simulink model "RBNN_NNT_timing_of_learning_1layerRBNN_openloop"  (R2019a)
settings: Solver=FixedStepAuto  StartTime=0.0  StopTime=inf  FixedStep=0.000001  RelTol=1e-3
libraries: dspstat3 x6, dspxfrm3 x1
(part 3 of 3)

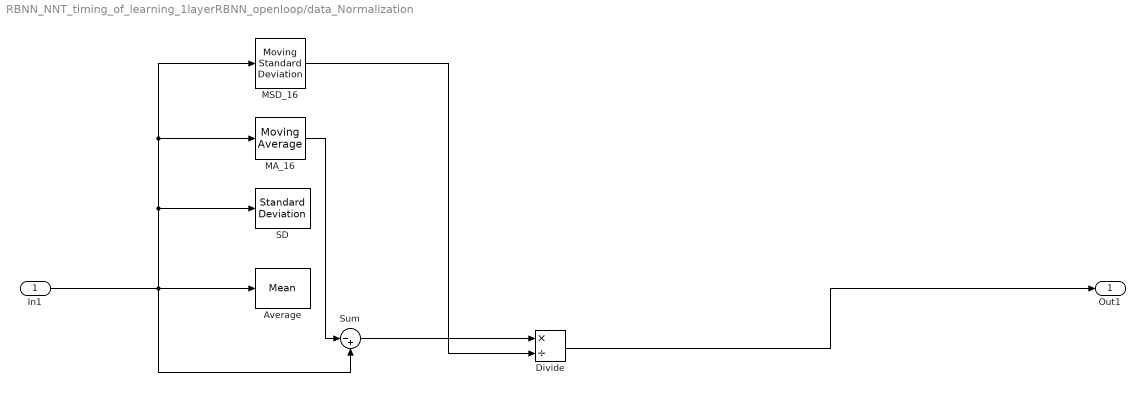
== system RBNN_NNT_timing_of_learning_1layerRBNN_openloop/data_Normalization ==
  In1 : Inport
  Average : dspstat3/Mean  run=on  reset_popup=None  directionMode=Each column  dimension=1  roiEnable=off  roiType=Rectangles  roiPortion=Entire ROI  roiOutput=Individual statistics for each ROI  roiFlag=off  roundingMode=Floor  overflowMode=off  outputDataTypeStr=Inherit: Same as accumulator  outputMin=[]  outputMax=[]  outputLastDataTypeStr=Inherit: Same as accumulator
  Divide : Product  Inputs=*/
  MA_16 : dspstat3/Moving Average  Method=Sliding window  ForgettingFactorPort=off  SpecifyWindowLength=on  WindowLength=4  ForgettingFactor=0.9  SimulateUsing=Code generation
  MSD_16 : dspstat3/Moving Standard Deviation  Method=Sliding window  ForgettingFactorPort=off  SpecifyWindowLength=on  WindowLength=4  ForgettingFactor=0.9  SimulateUsing=Code generation
      settings: SourceProductName=DSP System Toolbox  SourceProductBaseCode=DS
  SD : dspstat3/Standard Deviation  run=on  directionMode=Each column  dimension=1  reset_popup=None  roiEnable=off  roiType=Rectangles  roiPortion=Entire ROI  roiOutput=Individual statistics for each ROI  roiFlag=off
      settings: SourceProductName=DSP System Toolbox  SourceProductBaseCode=DS
  Sum : Sum  Inputs=|-+
  Out1 : Outport
  wires:
  In1/1 -> Sum/2, SD/1, MA_16/1, MSD_16/1, Average/1
  Sum/1 -> Divide/1
  Divide/1 -> Out1/1
  MSD_16/1 -> Divide/2
  MA_16/1 -> Sum/1

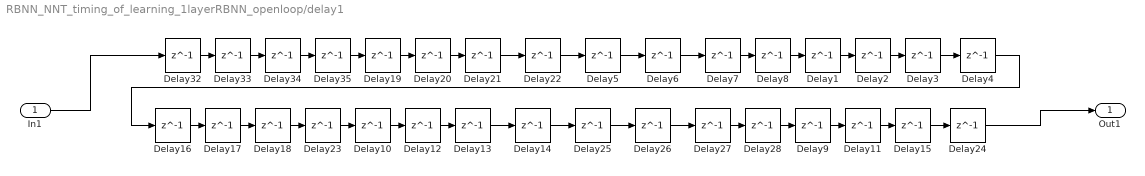
== system RBNN_NNT_timing_of_learning_1layerRBNN_openloop/delay1 ==
  In1 : Inport
  Delay{1..28,32..35} (32 alike) : Delay  DelayLength=1  InitialCondition=0
  Out1 : Outport
  wires:
  Delay34/1 -> Delay35/1
  Delay35/1 -> Delay19/1
  Delay33/1 -> Delay34/1
  Delay20/1 -> Delay21/1
  Delay21/1 -> Delay22/1
  Delay19/1 -> Delay20/1
  Delay32/1 -> Delay33/1
  Delay7/1 -> Delay8/1
  Delay8/1 -> Delay1/1
  Delay6/1 -> Delay7/1
  Delay2/1 -> Delay3/1
  Delay3/1 -> Delay4/1
  Delay1/1 -> Delay2/1
  Delay5/1 -> Delay6/1
  Delay22/1 -> Delay5/1
  Delay18/1 -> Delay23/1
  Delay15/1 -> Delay24/1
  Delay10/1 -> Delay12/1
  Delay17/1 -> Delay18/1
  Delay16/1 -> Delay17/1
  Delay13/1 -> Delay14/1
  Delay25/1 -> Delay26/1
  Delay27/1 -> Delay28/1
  Delay28/1 -> Delay9/1
  Delay14/1 -> Delay25/1
  Delay11/1 -> Delay15/1
  Delay26/1 -> Delay27/1
  Delay9/1 -> Delay11/1
  Delay23/1 -> Delay10/1
  Delay12/1 -> Delay13/1
  Delay4/1 -> Delay16/1
  Delay24/1 -> Out1/1
  In1/1 -> Delay32/1

== matlab function RBNN_NNT_timing_of_learning_1layerRBNN_openloop/NNT_O32 ==
  settings: sampleTime=0.125
  data: X0 input; X1 input; X2 input; X3 input; X4 input; X5 input; X6 input; X7 input; X8 input; X9 input; X10 input; X11 input; X12 input; X13 input; X14 input; X15 input; df input; y output; cost output; stop input; alpha_l input; a input
function [y,cost] = NN(X0,X1,X2,X3,X4,X5,X6,X7,X8,X9,X10,X11,X12,X13,X14,X15,df,stop,alpha_l,a)

%This is a generalised code for 2 layer - multiple input-single output network.
% to alter the network (1) "change layer's size" in layer declaration below (2) the function
%input and output above and (3) Input matrix creation. (4) change inputs in
%simulink design

alpha = alpha_l;

%(1)layer decalration

layer_0= 17;  % make it "16 + external_input's size"
layer_1=32;
layer_2 =1;


%(2) is above in function block

%(3)parameter intialisation
v=[X0 X1 X2 X3 X4 X5 X6 X7 X8 X9 X10 X11 X12 X13 X14 X15 transpose(a)];

%Do not alter the code below. The below implementaion is generalised for
%multiple input and single output, 2 layer neural network. 


persistent w1 w2;
persistent a1 a2;
persistent J; 
persistent v_old; 

if isempty(a1)
    a1= zeros(layer_1,1);
end

if isempty(a2)
    a2= zeros(layer_2,1);
end


if isempty(J)
    J= 0;
end
if isempty(v_old)
    v_old= zeros(1,layer_0);
end



if isempty(w1)
       w1=randn(layer_1,layer_0);
end
if isempty(w2)
       w2=randn(layer_2,layer_1);
end

%BackProp:
if stop==0
dz2=a2.*(1-a2)*df*-1;
dw2=dz2*transpose(a1);
dz1=(a1.*(1-a1)).*(w2'*dz2);
%dz1=a1.*(1-a1)*dz2;
dw1=dz1*v;
w2=w2 + alpha*dw2;
w1=w1 + alpha*dw1;
v_old=v;
end 

%forward propogation
z1=w1*v';
a1= (1./(1+exp(-z1)));
an1=a1-0.5;
z2=w2*an1;
a2= (1./(1+exp(-z2)));
an2=a2-0.5;
cost=1/2*df^2;

%output assignment
y=an2;


end

== matlab function RBNN_NNT_timing_of_learning_1layerRBNN_openloop/NN_RBNN_NN ==
  settings: sampleTime=0.01
  data: u1 input; df input; F input; u2 input; nn_op output; weights output; cost output; z1_out output; stop input; alp input; grad output; df_out output; del_weights output
function [nn_op,weights,cost,z1_out,grad,df_out,del_weights]   = NN(u1,df,F,u2,stop,alp)

persistent w1 ;
persistent vy;
persistent g1 ;
persistent itr;
persistent J;
persistent del_w1 ;
persistent mult1 ;
persistent memory_alloc_flag;
persistent n;

%%
%%%%%%----------------------------------------------------------------------------%%%%%
%Hyper-parameter & other tunable part of code

M=16;   %declare batch size of training (It will also be equal to number of input in our case as we are using DFT)
E=1;    % size of external associative input

%layer declaration
layer_1=16;
      % Output layer must match with number of rezonators declared in rezonator function

%learning rate. Currently reading from input pin 
alpha = alp;

%others
input_layer =M+E;       %layer_0
output_layer=layer_1;

% weight Intialisation 
if isempty(w1)
       w1=randn(input_layer,layer_1)*0.1;
end


%%%%%---------------------------------------------------------------------------------%%%%%

%%

%synchronising clock
if isempty(n)
        n = 0; end
n=n+1;

%%
%Allocation of variables that will be used during runtime( one time execution code) 
if isempty(memory_alloc_flag)
        memory_alloc_flag = 0; 
end
if isempty(mult1)
       mult1=zeros(layer_1,layer_1*input_layer); 
end
if isempty(vy)
       vy=zeros(input_layer,M); 
end

if memory_alloc_flag==0
 %write memory allocation for looped code here.It runs once and store it in memory.  
 mult1=[];
  for iteration =1:layer_1
   mult1=[mult1;[zeros(1,(iteration-1)*input_layer) ones(1,input_layer) zeros(1,(layer_1-iteration)*input_layer)]];
  end
  
 %{
 for k= 1:input_layer
    for j = 1:M 
        if k<=(M/2)+1 && k>=1
            vy(k,j)=0;
        elseif k<=M && k>=(M/2)+1
            vy(k,j)=0;
        elseif k>M
            vy(k,j)=0;     
        end
    end
 end
  %}
 memory_alloc_flag=1; 
end

%%
%============All other Initiaisation =========================>

%Initialisation of delta of weight storage
if isempty(del_w1)
    del_w1=zeros(1,input_layer*layer_1);
end


%Intialising iteration number & cost value. 
if isempty(itr)
    itr=0;
end
if isempty(J)
    J=0;
end


%gradient initialisation(in matrix form)
if isempty(g1)
    g1= zeros(M,input_layer*layer_1);   
end


%%
%Input vector creation code block
%x_in = [real(u1(1:(size(u1,2)/2)+1)) imag(u1(1:(size(u1,2)/2)-1))];
x_in=u1';
v=transpose([x_in transpose(u2)]);

%%
%RBNN core vectorised algorithm implementation 

%--------------->forward propogation ------------>

z1=w1'*v ;
a1=(1./(1+exp(-z1)));
an1=(a1-0.5);

%-------------> Backward Propogation -------->

%calculation of Nv:
da1_z1=a1.*(1-a1);
dn_a1=w1'.*repmat(da1_z1,1,size(v,1));
 

%calculation of aD, A & B 
aD=transpose(F)*dn_a1*vy;
A=[aD;eye(M-1) zeros(M-1,1)];
B=[transpose(F) ; zeros(M-1,size(F,1))]; 

%calculation of Nw(diff of N(v,w) wrt each weights)
dIn_1= da1_z1*transpose(v);
dn_w1=repmat(dIn_1,1,layer_1).* mult1;


%gradient updation

g1=A*g1+B*dn_w1;

%Training & updation only once in a batch(batch size=M,n=Overall counter) 
if mod(n,M)==0 && stop==0
%if stop==0
    %del_w1 =alpha*df(1)*1*g1(1,:) ;
    del_w1 =alpha*df*1*g1/M ;
    del_w_reshaped1= reshape(del_w1,[input_layer,layer_1]);
    w1=w1+ del_w_reshaped1;
    itr=itr+1;
    %J= sum(df.^2,'all')/(2*M);
end

J= 1/2*df(1).^2;
%For logging & visulisation purpose
cost=J;
weights=w1;
z1_out=z1;
grad=g1(1,:);
df_out=df(1);
del_weights=del_w1;
%NN output assignment
nn_op=an1;


end

== matlab function RBNN_NNT_timing_of_learning_1layerRBNN_openloop/buffer_of_op_fft ==
  data: output_difference_vector output size=[1,16]; output_fft output size=[1,16]; dif_ip input; rbnn_output input
function [output_difference_vector,output_fft] = difBuffer(dif_ip,rbnn_output)                      

 sz=16;                       % size of the dft 
 
 persistent a;
 persistent b;
 if isempty(b)
  b= zeros(1,sz);
 end
 if isempty(a)
  a= zeros(1,sz);
 end
 
 
  a= circshift(a,1);
  a(1)=dif_ip;
  b= circshift(b,1);
  b(1)=rbnn_output;

 output_difference_vector=a; 
 output_fft=1/sz*fft(b); 
end

== matlab function RBNN_NNT_timing_of_learning_1layerRBNN_openloop/NNT_O64 ==
  settings: sampleTime=0.125
  data: X0 input; X1 input; X2 input; X3 input; X4 input; X5 input; X6 input; X7 input; X8 input; X9 input; X10 input; X11 input; X12 input; X13 input; X14 input; X15 input; df input; y output; cost output; stop input; alpha_l input; a input
function [y,cost] = NN(X0,X1,X2,X3,X4,X5,X6,X7,X8,X9,X10,X11,X12,X13,X14,X15,df,stop,alpha_l,a)

%This is a generalised code for 2 layer - multiple input-single output network.
% to alter the network (1) "change layer's size" in layer declaration below (2) the function
%input and output above and (3) Input matrix creation. (4) change inputs in
%simulink design

alpha = alpha_l;

%(1)layer decalration

layer_0= 17;  % make it "16 + external_input's size"
layer_1=64;
layer_2 =1;


%(2) is above in function block

%(3)parameter intialisation
v=[X0 X1 X2 X3 X4 X5 X6 X7 X8 X9 X10 X11 X12 X13 X14 X15 transpose(a)];

%Do not alter the code below. The below implementaion is generalised for
%multiple input and single output, 2 layer neural network. 


persistent w1 w2;
persistent a1 a2;
persistent J; 
persistent v_old; 

if isempty(a1)
    a1= zeros(layer_1,1);
end

if isempty(a2)
    a2= zeros(layer_2,1);
end


if isempty(J)
    J= 0;
end
if isempty(v_old)
    v_old= zeros(1,layer_0);
end



if isempty(w1)
       w1=randn(layer_1,layer_0);
end
if isempty(w2)
       w2=randn(layer_2,layer_1);
end

%BackProp:
if stop==0
dz2=a2.*(1-a2)*df*-1;
dw2=dz2*transpose(a1);
dz1=(a1.*(1-a1)).*(w2'*dz2);
%dz1=a1.*(1-a1)*dz2;
dw1=dz1*v;
w2=w2 + alpha*dw2;
w1=w1 + alpha*dw1;
v_old=v;
end 

%forward propogation
z1=w1*v';
a1= (1./(1+exp(-z1)));
an1=a1-0.5;
z2=w2*an1;
a2= (1./(1+exp(-z2)));
an2=a2-0.5;
cost=1/2*df^2;

%output assignment
y=an2;


end

== matlab function RBNN_NNT_timing_of_learning_1layerRBNN_openloop/NNT_O16 ==
  settings: sampleTime=0.125
  data: X0 input; X1 input; X2 input; X3 input; X4 input; X5 input; X6 input; X7 input; X8 input; X9 input; X10 input; X11 input; X12 input; X13 input; X14 input; X15 input; df input; y output; cost output; stop input; alpha_l input; a input
function [y,cost] = NN(X0,X1,X2,X3,X4,X5,X6,X7,X8,X9,X10,X11,X12,X13,X14,X15,df,stop,alpha_l,a)

%This is a generalised code for 2 layer - multiple input-single output network.
% to alter the network (1) "change layer's size" in layer declaration below (2) the function
%input and output above and (3) Input matrix creation. (4) change inputs in
%simulink design

alpha = alpha_l;

%(1)layer decalration

layer_0= 17;  % make it "16 + external_input's size"
layer_1=16;
layer_2 =1;


%(2) is above in function block

%(3)parameter intialisation
v=[X0 X1 X2 X3 X4 X5 X6 X7 X8 X9 X10 X11 X12 X13 X14 X15 transpose(a)];

%Do not alter the code below. The below implementaion is generalised for
%multiple input and single output, 2 layer neural network. 


persistent w1 w2;
persistent a1 a2;
persistent J; 
persistent v_old; 

if isempty(a1)
    a1= zeros(layer_1,1);
end

if isempty(a2)
    a2= zeros(layer_2,1);
end


if isempty(J)
    J= 0;
end
if isempty(v_old)
    v_old= zeros(1,layer_0);
end



if isempty(w1)
       w1=randn(layer_1,layer_0);
end
if isempty(w2)
       w2=randn(layer_2,layer_1);
end

%BackProp:
if stop==0
dz2=a2.*(1-a2)*df*-1;
dw2=dz2*transpose(a1);
dz1=(a1.*(1-a1)).*(w2'*dz2);
%dz1=a1.*(1-a1)*dz2;
dw1=dz1*v;
w2=w2 + alpha*dw2;
w1=w1 + alpha*dw1;
v_old=v;
end 

%forward propogation
z1=w1*v';
a1= (1./(1+exp(-z1)));
an1=a1-0.5;
z2=w2*an1;
a2= (1./(1+exp(-z2)));
an2=a2-0.5;
cost=1/2*df^2;

%output assignment
y=an2;


end

== matlab function RBNN_NNT_timing_of_learning_1layerRBNN_openloop/software_rezonator ==
  data: signalz input; reconstructed_signal output; Fn output size=16
function [reconstructed_signal,Fn]   = rezonator(signalz)

persistent numberofrezonator;
persistent g c bfr_rezo_sm aft_delay dft_out;
persistent out signal_dif;
persistent n;
persistent memory_alloc_flag;


%assign the number of rezonator here. For configuring it for higher order
%rezonator  we need to change (1) 'numberofrezonaotor' variable
if isempty(numberofrezonator)
        numberofrezonator = 16;   %here 16 parallel rezonators
end
N=16;
%Initialisation of memory allocations/variables ====> 
if isempty(memory_alloc_flag)
        memory_alloc_flag = 0; 
end
if isempty(g)
       g=zeros(numberofrezonator,numberofrezonator,'like',0i); 
end
if isempty(c)
       c=zeros(numberofrezonator,numberofrezonator,'like',0i); 
end
if memory_alloc_flag==0
 for i=0:numberofrezonator-1
  for j= 0:numberofrezonator-1
   g(i+1,j+1)=1/numberofrezonator*(exp(-1i*2*pi*i*j/numberofrezonator));
   c(i+1,j+1)=(exp(1i*2*pi*i*j/numberofrezonator));
  end 
 end
 memory_alloc_flag=1;
end


%Initialisation of variables  =====> 
if isempty(n)
        n = 0;   
end 
if isempty(out)
  out=0+0i;
end
if isempty(signal_dif)
  signal_dif=0+0i;
end
if isempty(bfr_rezo_sm)
  bfr_rezo_sm=repmat(0+0i,numberofrezonator,1);
end
if isempty(aft_delay)
  aft_delay=repmat(0+0i,numberofrezonator,1);
end
if isempty(dft_out)
  dft_out=repmat(0+0i,numberofrezonator,1);
end

%creating cycle of rotation for selection of correct column of g & c.
cycle=mod(n,numberofrezonator);

%resonator core -----------------------------> 
dft_out=c(:,cycle+1).*aft_delay;
out= sum(dft_out,1);
signal_dif=signalz-out;
bfr_rezo_sm=g(:,cycle+1).*signal_dif;

%counting the counter
n=n+1;

% output assignment ------------------>
reconstructed_signal=out;
dft=aft_delay; 
%N=size(dft,1);
a=1:1:N/2-1;
b=N/2+1:1:N-1;
dft_trans=transpose(dft);
Fn=transpose([real(dft_trans(1)) 2*(real(dft_trans(2:N/2)).*cos(2*pi*a*n/N)-imag(dft_trans(2:N/2)).*sin(2*pi*a*n/N)) -1^n*real(dft_trans(N/2+1)) -2*(imag(dft_trans(N/2+2:N)).*cos(2*pi*b*n/N)+real(dft_trans(N/2+2:N)).*sin(2*pi*b*n/N))]);
%--------output assignment over----------<

%final updation of buffer ------>>>>>>>>>>>>
aft_delay= aft_delay+bfr_rezo_sm; 
end

== matlab function RBNN_NNT_timing_of_learning_1layerRBNN_openloop/N_RBNN_output ==
  data: dft input; yn output; freq_char input
function yn = fcn(dft,freq_char)
yn=transpose(freq_char)*dft;
end

== matlab function RBNN_NNT_timing_of_learning_1layerRBNN_openloop/4. Training Signal Generation ==
  data: pulse output
function pulse   = fcn()
M=16;

persistent cnt;
persistent n;
if isempty(cnt)
    cnt=0;
end
if isempty(n)
    n=0;
end
n=n+1;
if mod(n,M)==0
     cnt=cnt+1;
 end
 pulse = mod(cnt,2);

end
